simulink model "NumSim_standard_eVTOL"  (R2024b)
settings: Solver=ode14x  StartTime=0.0  StopTime=250  FixedStep=0.005  RelTol=1e-3
values from neighbouring files (symbols this model uses):
  aDl =     [initdata.mat]
  aDr =     [initdata.mat]
  aDyn =     [initdata.mat]
  Airport = init_airport('PHNL')    [initdata_HIL_eVTOL.m]
  aLat =     [initdata.mat]
  aLon =     [initdata.mat]
  D = Prop.D    [EOM_dt_MC.m]    (also in EOM_get_alf_dt_de_prop_evtol.m = CD * QS)
  dt0 = X(2)    [EOM_get_alf_dt_de_prop_evtol.m]    (also in initdata.mat = 0.258252593971; initdata_HIL_eVTOL.m = EOM_dt_MC)
  EAS0 = TAS0 / EAS2TAS    [initdata_HIL_eVTOL.m]
  FCS = init_FCS    [initdata_HIL_eVTOL.m]
  General = init_layoutdata    [EOM_dt_MC.m]    (also in build_optimized_CA.m; initdata.mat = ; initdata_HIL_eVTOL.m)
  h0 = Con(1)    [EOM_get_alf_dt_de_prop_evtol.m]    (also in initdata.mat = 450; initdata_HIL_eVTOL.m = 50)
  mass = Con(3)    [EOM_get_alf_dt_de_prop_evtol.m]    (also in initdata.mat = 2255.54; initdata_HIL_eVTOL.m = 7)
  Motor = init_motor_evtol    [EOM_dt_MC.m]    (also in initdata.mat = []; initdata_HIL_eVTOL.m)
  Prop = init_propeller_evtol_new    [EOM_dt_MC.m]    (also in initdata_HIL_eVTOL.m)
  R2D = 180/pi    (= 57.2957795131)    [EOM_get_alf_dt_de_prop_evtol.m]    (also in init_FCS.m; init_aerodata_evtol.m; init_airport.m; initdata.mat)
  theta0 = -0.0510981441662    [initdata.mat]
undefined symbols (not defined in the file or in its folder): A1, aDa, aDe, asbhl20env, B1, C1, de0, Earth, Environment, InitData, Kd, Kp, magnitude, Tc, WGS84
libraries: simulink_extras x26, simulink x18, slpidlib x14, vrlib x8, matrix_library x6, sharedutil x6, sharedtransform x5, aerolibwindfilters x4, aerolibatmos2 x3, aerolibobsolete x2, aerolibactuator x2, aerolibasang x2
(part 1 of 7)
settings Model: SimulationMode=accelerator  Creator=Administrator  LastModifiedBy=ZDB
settings SolverCC: EnableFixedStepZeroCrossing=on
settings OptimizationCC: ReuseModelBlockBuffer=off
settings DebuggingCC: UnconnectedInputMsg=warning  UnconnectedOutputMsg=warning  UnconnectedLineMsg=warning
settings ModelReferenceCC: EnableRefExpFcnMdlSchedulingChecks=on
settings RTWCC: GPUComputeCapability=3.5  DLArmComputeVersion=19.05

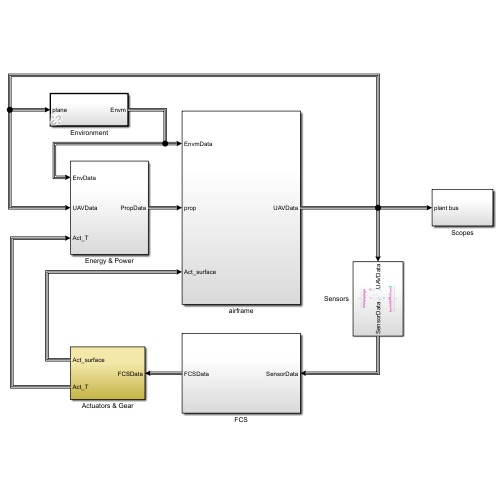
[thumbnail: Simulink's stored preview of the top-level diagram]
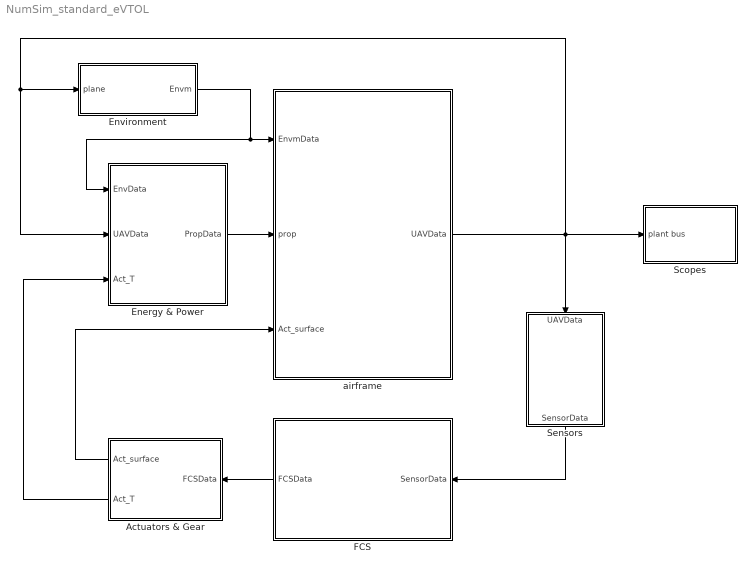
== system NumSim_standard_eVTOL ==
  Actuators & Gear : Subsystem
  Energy & Power : Subsystem
  Environment : Subsystem  AncestorBlock=asbhl20env/Environment  TreatAsAtomicUnit=on
      settings: LibrarySourceBlock=asbhl20env/Environment
  FCS : Subsystem
  Scopes : Subsystem
  Sensors : Subsystem
  airframe : Subsystem
  wires:
  Energy & Power/1(PropData) -> airframe/2(prop)
  Actuators & Gear/2(Act_T) -> Energy & Power/3(Act_T)
  airframe/1(UAVData) -> Energy & Power/2(UAVData), Environment/1(plane), Sensors/1(UAVData), Scopes/1(plant bus)
  Actuators & Gear/1(Act_surface) -> airframe/3(Act_surface)
  Environment/1(Envm) -> Energy & Power/1(EnvData), airframe/1(EnvmData)
  FCS/1(FCSData) -> Actuators & Gear/1(FCSData)
  Sensors/1(SensorData) -> FCS/1(SensorData)

== system NumSim_standard_eVTOL/Actuators & Gear ==
  FCSData : Inport
  Bus Creator : BusCreator  Inputs=3
  Bus Creator1 : BusCreator  Inputs=7
  Bus Selector : BusSelector  OutputSignals=ACTCMD.dl_cmd,ACTCMD.dt_final,ACTCMD.dr_cmd,ACTCMD.da_cmd,SensorData.Va,FCSCMD.icmd
  Demux : Demux  Outputs=6
  Gain{,1..11} (12 alike) : Gain
  Gain12 : Gain  Gain=57.3
  Max : MinMax  Function=max  Inputs=2
  Mux : Mux  Inputs=3
  Radians to Degrees1 : simulink_extras/Transformations/Radians to Degrees
  Radians to Degrees2 : simulink_extras/Transformations/Radians to Degrees
  Radians to Degrees3 : simulink_extras/Transformations/Radians to Degrees
  Rate Limiter : RateLimiter  RisingSlewLimit=0.12  FallingSlewLimit=-0.2  SampleTimeMode=inherited
  Saturation1 : Saturate  UpperLimit=25/57.3  LowerLimit=-25/57.3
  Saturation2 : Saturate  UpperLimit=25/57.3  LowerLimit=-25/57.3
  Saturation3 : Saturate  UpperLimit=25/57.3  LowerLimit=-25/57.3
  Scope : Scope
  Scope1 : Scope
  Scope3 : Scope
  Selector : Selector  InputPortWidth=3  IndexOptions=Index vector (dialog)  Indices=2  OutputSizes=1
  Selector1 : Selector  InputPortWidth=3  IndexOptions=Index vector (dialog)  Indices=3  OutputSizes=1
  Selector2 : Selector  InputPortWidth=3  IndexOptions=Index vector (dialog)  Indices=1  OutputSizes=1
  To Workspace : ToWorkspace  VariableName=i  SaveFormat=Timeseries  SampleTime=-1
  control output FW : Scope  NumInputPorts=3
  i : Constant  Commented=on  Value=0
  safe i_min : Lookup_n-D  NumberOfTableDimensions=1  BreakpointsForDimension1=[0,2,3.5,5,8,11,13,16,19,20,21, 22,30]  Table=[1.22,1.19,1.13,1.05,0.96,0.84,0.7,0.52,0.31,0.14,0.04,0,0]  InternalRulePriority=Speed  RndMeth=Simplest
  theta_b : Constant  Commented=on  Value=72.43773 * pi / 180
  Act_surface : Outport  VectorParamsAs1DForOutWhenUnconnected=off
  Act_T : Outport  Port=2  VectorParamsAs1DForOutWhenUnconnected=off
  tag scope: i=global
  wires:
  Mux/1 -> Selector2/1, Selector/1, Selector1/1
  Bus Creator/1 -> Act_surface/1
  Selector2/1 -> Gain6/1
  Saturation1/1 -> Gain3/1
  Saturation2/1 -> Radians to Degrees1/1, Bus Creator/2  "dr"
  Saturation3/1 -> Radians to Degrees2/1, Bus Creator/3  "da"
  Gain3/1 -> Radians to Degrees3/1, Bus Creator/1  "dl"
  Selector1/1 -> Gain1/1
  Selector/1 -> Gain/1
  Radians to Degrees3/1 -> control output FW/1  "da"
  Radians to Degrees1/1 -> control output FW/2  "de"
  Radians to Degrees2/1 -> control output FW/3  "dr"
  Gain/1 -> Gain4/1  "dr"
  Gain1/1 -> Gain5/1  "da"
  Gain4/1 -> Saturation2/1
  Gain5/1 -> Saturation3/1
  Bus Creator1/1 -> Act_T/1
  Gain6/1 -> Saturation1/1  "dl"
  FCSData/1 -> Bus Selector/1
  Bus Selector/1 -> Mux/1  "<dl_cmd>"
  Bus Selector/3 -> Mux/2  "<dr_cmd>"
  Bus Selector/4 -> Mux/3  "<da_cmd>"
  Gain2/1 -> Scope/1, Bus Creator1/1  "dt_1"
  Gain7/1 -> Scope3/1, Bus Creator1/2  "dt_2"
  Gain8/1 -> Bus Creator1/3  "dt_3"
  Gain9/1 -> Bus Creator1/4  "dt_4"
  Gain10/1 -> Bus Creator1/5  "dt_5"
  Gain11/1 -> Bus Creator1/6  "dt_6"
  Bus Selector/5 -> safe i_min/1  "<Va>"
  safe i_min/1 -> Max/2
  Max/1 -> Rate Limiter/1  "i"
  Bus Selector/6 -> Max/1  "<icmd>"
  Demux/1 -> Gain2/1
  Demux/2 -> Gain7/1
  Demux/3 -> Gain8/1
  Demux/4 -> Gain9/1
  Demux/5 -> Gain10/1
  Demux/6 -> Gain11/1
  Bus Selector/2 -> Demux/1  "<dt_final>"
  Rate Limiter/1 -> Gain12/1, Scope1/1, Bus Creator1/7, [i]  "i"
  Gain12/1 -> To Workspace/1

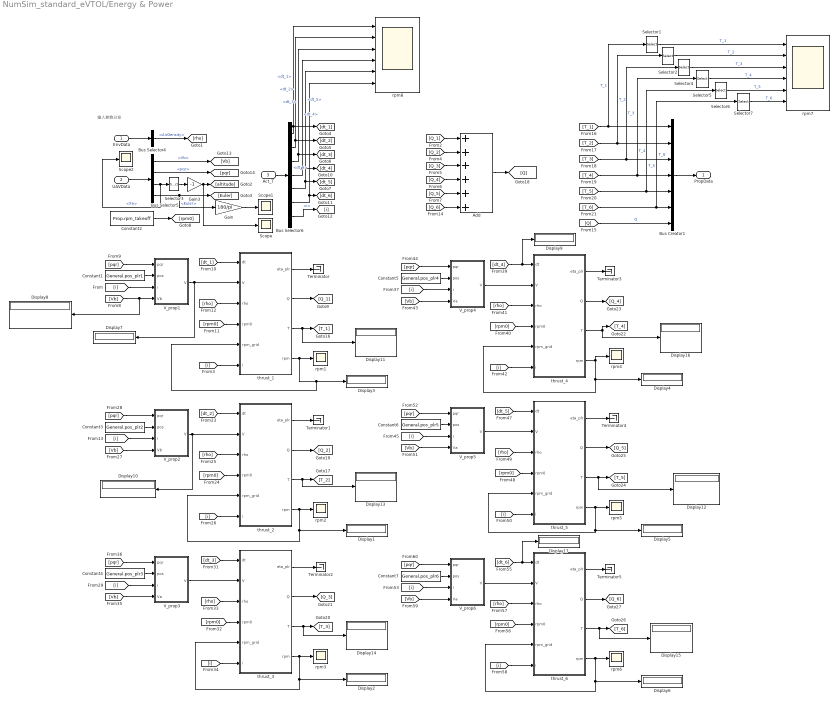
== system NumSim_standard_eVTOL/Energy & Power ==
  note: 输入参数分发
  EnvData : Inport
  UAVData : Inport  Port=2
  Act_T : Inport  Port=3
  Add : Sum  Inputs=++++++
  Bus Creator1 : BusCreator  Inputs=7
  Bus Selector4 : BusSelector  OutputSignals=AirDensity
  Bus Selector5 : BusSelector  OutputSignals=Vb,pqr,Xe,Euler
  Bus Selector6 : BusSelector  OutputSignals=dt_1,dt_2,dt_3,dt_4,dt_5,dt_6,i
  Constant1 : Constant  Value=General.pos_plr1
  Constant2 : Constant  Value=Prop.rpm_takeoff
  Constant3 : Constant  Value=General.pos_plr2
  Constant4 : Constant  Value=General.pos_plr3
  Constant5 : Constant  Value=General.pos_plr4
  Constant6 : Constant  Value=General.pos_plr5
  Constant7 : Constant  Value=General.pos_plr6
  Display{1..17} (17 alike) : Display
  Gain : Gain  Gain=180/pi
  Gain3 : Gain  Gain=-1
  Scope : Scope
  Scope1 : Scope
  Scope2 : Scope
  Selector{1..7} (7 alike) : Selector  InputPortWidth=3  IndexOptions=Index vector (dialog)  Indices=3  OutputSizes=1
  Terminator{,1..5} (6 alike) : Terminator
  V_prop1 : Subsystem
  V_prop2 : Subsystem
  V_prop3 : Subsystem
  V_prop4 : Subsystem
  V_prop5 : Subsystem
  V_prop6 : Subsystem
  rpm{1..6} (6 alike) : Scope
  rpm7 : Scope  NumInputPorts=6
  rpm8 : Scope  NumInputPorts=6
  thrust_1 : Subsystem
  thrust_2 : Subsystem
  thrust_3 : Subsystem
  thrust_4 : Subsystem
  thrust_5 : Subsystem
  thrust_6 : Subsystem
  PropData : Outport  VectorParamsAs1DForOutWhenUnconnected=off
  wires:
  Act_T/1 -> Bus Selector6/1
  [dt_1] -> thrust_1/1(dt)
  Constant1/1 -> V_prop1/2(pos)
  [rho] -> thrust_1/3(rho)
  [rpm0] -> thrust_1/4(rpm0)
  thrust_1/1(eta_plr) -> Terminator/1
  [pqr] -> V_prop1/1(pqr)
  [Vb] -> Display8/1, V_prop1/4(Vb)
  EnvData/1 -> Bus Selector4/1
  Bus Selector4/1 -> [rho]  "<AirDensity>"
  Bus Selector5/2 -> [pqr]  "<pqr>"
  Selector3/1 -> Gain3/1
  UAVData/1 -> Bus Selector5/1
  Bus Selector5/4 -> Gain/1, [Euler]  "<Euler>"
  Bus Selector5/1 -> [Vb]  "<Vb>"
  Bus Selector5/3 -> Scope2/1, Selector3/1  "<Xe>"
  Bus Selector6/1 -> rpm8/1, [dt_1]  "<dt_1>"
  Bus Selector6/5 -> [dt_5], rpm8/5  "<dt_5>"
  Bus Selector6/3 -> [dt_3], rpm8/3  "<dt_3>"
  Bus Selector6/2 -> [dt_2], rpm8/2  "<dt_2>"
  V_prop1/1(V) -> thrust_1/2(V), Display7/1
  [i] -> V_prop1/3(i)
  Constant2/1 -> [rpm0]
  thrust_1/4(rpm) -> thrust_1/5(rpm_grid), Display3/1, rpm1/1
  thrust_1/2(Q) -> [Q_1]
  Bus Selector6/4 -> [dt_4], rpm8/4  "<dt_4>"
  Bus Selector6/6 -> rpm8/6, [dt_6]  "<dt_6>"
  Bus Selector6/7 -> [i]  "<i>"
  [i] -> thrust_1/6(i)
  thrust_1/3(T) -> Display11/1, [T_1]
  [Q_1] -> Add/1
  [Q_6] -> Add/6
  [Q_5] -> Add/5
  [Q_4] -> Add/4
  [Q_3] -> Add/3
  [Q_2] -> Add/2
  Add/1 -> [Q]
  [Q] -> Bus Creator1/7  "Q"
  [T_1] -> Selector1/1, Bus Creator1/1  "T_1"
  [T_2] -> Selector2/1, Bus Creator1/2  "T_2"
  [T_3] -> Bus Creator1/3, Selector4/1  "T_3"
  [T_4] -> Bus Creator1/4, Selector5/1  "T_4"
  [T_5] -> Bus Creator1/5, Selector6/1  "T_5"
  [T_6] -> Bus Creator1/6, Selector7/1  "T_6"
  Bus Creator1/1 -> PropData/1
  thrust_2/4(rpm) -> rpm2/1, thrust_2/5(rpm_grid), Display1/1
  Constant3/1 -> V_prop2/2(pos)
  [dt_2] -> thrust_2/1(dt)
  V_prop2/1(V) -> Display10/1, thrust_2/2(V)
  thrust_2/2(Q) -> [Q_2]
  thrust_2/1(eta_plr) -> Terminator1/1
  [i] -> V_prop2/3(i)
  thrust_2/3(T) -> [T_2], Display13/1
  [rpm0] -> thrust_2/4(rpm0)
  [Vb] -> V_prop2/4(Vb)
  [pqr] -> V_prop2/1(pqr)
  [i] -> thrust_2/6(i)
  [rho] -> thrust_2/3(rho)
  [rho] -> thrust_3/3(rho)
  [pqr] -> V_prop3/1(pqr)
  [Vb] -> V_prop3/4(Va)
  [i] -> V_prop3/3(i)
  thrust_3/2(Q) -> [Q_3]
  V_prop3/1(V) -> thrust_3/2(V)
  [rpm0] -> thrust_3/4(rpm0)
  [dt_3] -> thrust_3/1(dt)
  thrust_3/4(rpm) -> thrust_3/5(rpm_grid), Display2/1, rpm3/1
  Constant4/1 -> V_prop3/2(pos)
  thrust_3/1(eta_plr) -> Terminator2/1
  [i] -> thrust_3/6(i)
  thrust_3/3(T) -> Display14/1, [T_3]
  [i] -> thrust_4/6(i)
  thrust_4/4(rpm) -> rpm4/1, thrust_4/5(rpm_grid), Display4/1
  Constant5/1 -> V_prop4/2(pos)
  thrust_4/1(eta_plr) -> Terminator3/1
  thrust_4/3(T) -> [T_4], Display16/1
  [dt_4] -> Display9/1, thrust_4/1(dt)
  V_prop4/1(V) -> thrust_4/2(V)
  [rpm0] -> thrust_4/4(rpm0)
  [i] -> V_prop4/3(i)
  [Vb] -> V_prop4/4(Va)
  [pqr] -> V_prop4/1(pqr)
  [rho] -> thrust_4/3(rho)
  thrust_4/2(Q) -> [Q_4]
  thrust_5/2(Q) -> [Q_5]
  thrust_5/3(T) -> Display12/1, [T_5]
  [rho] -> thrust_5/3(rho)
  [pqr] -> V_prop5/1(pqr)
  [rpm0] -> thrust_5/4(rpm0)
  Constant6/1 -> V_prop5/2(pos)
  thrust_5/1(eta_plr) -> Terminator4/1
  [dt_5] -> thrust_5/1(dt)
  [i] -> V_prop5/3(i)
  V_prop5/1(V) -> thrust_5/2(V)
  [i] -> thrust_5/6(i)
  thrust_5/4(rpm) -> thrust_5/5(rpm_grid), Display5/1, rpm5/1
  [Vb] -> V_prop5/4(Va)
  [i] -> V_prop6/3(i)
  [Vb] -> V_prop6/4(Va)
  thrust_6/1(eta_plr) -> Terminator5/1
  V_prop6/1(V) -> thrust_6/2(V)
  [dt_6] -> Display17/1, thrust_6/1(dt)
  thrust_6/4(rpm) -> thrust_6/5(rpm_grid), Display6/1, rpm6/1
  thrust_6/2(Q) -> [Q_6]
  thrust_6/3(T) -> Display15/1, [T_6]
  Constant7/1 -> V_prop6/2(pos)
  [rho] -> thrust_6/3(rho)
  [pqr] -> V_prop6/1(pqr)
  [rpm0] -> thrust_6/4(rpm0)
  [i] -> thrust_6/6(i)
  Selector1/1 -> rpm7/1  "T_1"
  Selector2/1 -> rpm7/2  "T_2"
  Selector4/1 -> rpm7/3  "T_3"
  Selector5/1 -> rpm7/4  "T_4"
  Selector6/1 -> rpm7/5  "T_5"
  Selector7/1 -> rpm7/6  "T_6"
  Gain3/1 -> Scope/1, [altitude]
  Gain/1 -> Scope1/1

== system NumSim_standard_eVTOL/Environment ==
  plane : Inport
  Bus Creator : BusCreator  Inputs=8
  Bus Selector : BusSelector  OutputSignals=Xe,Ve,DCM_be
  COESA Atmosphere Model : aerolibatmos2/COESA Atmosphere Model  units=Metric (MKS)  spec=1976 COESA-extended U.S. Standard Atmosphere  model=Profile  profile_var=High temperature  profile_percent=1%  profile_alt=5 km (16404 ft)  envelope_var=High temperature  envelope_percent=1%  action=Warning
  Height : Selector  InputPortWidth=3  IndexOptions=Index vector (dialog)  Indices=[3]  OutputSizes=1
  Latitude : Constant  Value=40
  Terrain : Subsystem
  WGS84 Gravity Model : aerolibobsolete/WGS84 Gravity Model  model=WGS84 Taylor Series  units=Metric (MKS)  no_atmos=on  precessing=on  month=February  day=1  year=2000  no_centrifugal=on  action=None
  Wind Models : Subsystem
  x : Selector  InputPortWidth=3  IndexOptions=Index vector (dialog)  Indices=1  OutputSizes=1
  z-->h : Abs
  Envm : Outport  InitialOutput=0  VectorParamsAs1DForOutWhenUnconnected=off
  wires:
  COESA Atmosphere Model/4 -> Bus Creator/7  "AirDensity"
  COESA Atmosphere Model/2 -> Bus Creator/5  "a"
  COESA Atmosphere Model/3 -> Bus Creator/6  "Po"
  COESA Atmosphere Model/1 -> Bus Creator/4  "To"
  Height/1 -> z-->h/1
  Bus Creator/1 -> Envm/1  "EnvmData"
  plane/1 -> Bus Selector/1
  z-->h/1 -> COESA Atmosphere Model/1, WGS84 Gravity Model/1, Wind Models/3(Altitude)
  Bus Selector/1 -> x/1, Terrain/1(Xe), Height/1  "<Xe>"
  Bus Selector/2 -> Wind Models/2(Ve)  "<Ve>"
  Bus Selector/3 -> Wind Models/4(DCM)  "<DCM_be>"
  Latitude/1 -> WGS84 Gravity Model/2
  WGS84 Gravity Model/1 -> Bus Creator/8  "g"
  Terrain/1(hground) -> Bus Creator/1  "hground"
  Wind Models/1(ug,vg,wg1) -> Bus Creator/2
  Wind Models/2(pg,qg,rg1) -> Bus Creator/3
  x/1 -> Wind Models/1(Xe_x)

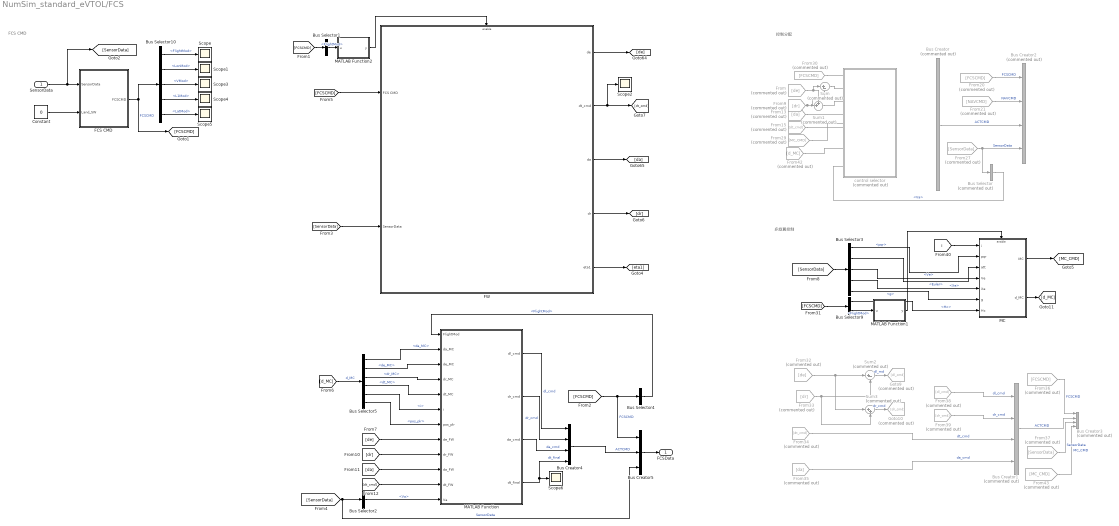
== system NumSim_standard_eVTOL/FCS ==
  note: 控制分配
  note: 多旋翼控制
  note: FCS CMD
  SensorData : Inport
  Bus Creator{,1..3} (4 alike) : BusCreator  Commented=on  Inputs=4
  Bus Creator4 : BusCreator  Inputs=4
  Bus Creator5 : BusCreator  Inputs=3
  Bus Selector : BusSelector  Commented=on  OutputSignals=Va
  Bus Selector1 : BusSelector  OutputSignals=FlightMod
  Bus Selector10 : BusSelector  OutputSignals=FlightMod,LonMod,VMod,L1Mod,LatMod
  Bus Selector2 : BusSelector  OutputSignals=Va
  Bus Selector3 : BusSelector  OutputSignals=pqr,Euler,Ve,Xe,g
  Bus Selector4 : BusSelector  OutputSignals=FlightMod
  Bus Selector5 : BusSelector  OutputSignals=da_MC,de_MC,dr_MC,dt_MC,i,pos_plr
  Bus Selector9 : BusSelector  OutputSignals=Hc,FlightMod
  Constant : Constant  Value=0
  FCS CMD : Subsystem
  FW : Subsystem
  From : From  Commented=on  GotoTag=de
  From13 : From  Commented=on  GotoTag=da
  From15 : From  Commented=on  GotoTag=dt_cmd
  From20 : From  Commented=on  GotoTag=FCSCMD
      settings: CloseFcn=tagdialog Close
  From21 : From  Commented=on  GotoTag=NAVCMD
      settings: CloseFcn=tagdialog Close
  From27 : From  Commented=on  GotoTag=SensorData
  From29 : From  Commented=on  GotoTag=MC_CMD
  From30 : From  Commented=on  GotoTag=FCSCMD
      settings: CloseFcn=tagdialog Close
  From32 : From  Commented=on  GotoTag=de
  From33 : From  Commented=on  GotoTag=dr
  From34 : From  Commented=on  GotoTag=dt_cmd
  From35 : From  Commented=on  GotoTag=da
  From36 : From  Commented=on  GotoTag=FCSCMD
  From37 : From  Commented=on  GotoTag=SensorData
  From38 : From  Commented=on  GotoTag=dl_cmd
  From39 : From  Commented=on  GotoTag=dr_cmd
  From42 : From  Commented=on  GotoTag=d_MC
  From43 : From  Commented=on  GotoTag=MC_CMD
  From9 : From  Commented=on  GotoTag=dr
  Goto10 : Goto  Commented=on  GotoTag=dr_cmd
  Goto9 : Goto  Commented=on  GotoTag=dl_cmd
  MATLAB Function : MATLAB Function  TreatAsAtomicUnit=on
  MATLAB Function1 : MATLAB Function  TreatAsAtomicUnit=on
  MATLAB Function2 : MATLAB Function  TreatAsAtomicUnit=on
  MC : Subsystem
  Scope{,1..6} (7 alike) : Scope
  Sum : Sum  Commented=on  Inputs=|+-
  Sum1 : Sum  Commented=on  Inputs=++|
  Sum2 : Sum  Commented=on  Inputs=|+-
  Sum3 : Sum  Commented=on  Inputs=|++
  control selector : Subsystem  Commented=on
  FCSData : Outport  VectorParamsAs1DForOutWhenUnconnected=off
  wires:
  Bus Creator/1 -> Bus Creator2/3  "ACTCMD"
  SensorData/1 -> FCS CMD/1(SensorData), [SensorData]
  FCS CMD/1(FCSCMD) -> Bus Selector10/1, [FCSCMD]  "FCSCMD"
  From20/1 -> Bus Creator2/1  "FCSCMD"
  From21/1 -> Bus Creator2/2  "NAVCMD"
  From30/1 -> ?
  [SensorData] -> Bus Selector3/1
  Bus Selector3/1 -> MC/2(pqr)  "<pqr>"
  Bus Selector3/2 -> MC/3(att)  "<Euler>"
  Bus Selector3/3 -> MC/4(Ve)  "<Ve>"
  Bus Selector3/4 -> MC/5(Xe)  "<Xe>"
  Constant/1 -> FCS CMD/2(Land_SW)
  MC/1(MC) -> [MC_CMD]
  Bus Selector3/5 -> MC/6(g)  "<g>"
  From/1 -> Sum1/1, Sum/1
  From9/1 -> Sum/2, Sum1/2
  Sum/1 -> ?
  Sum1/1 -> ?
  From13/1 -> ?
  From15/1 -> ?
  From27/1 -> Bus Selector/1, Bus Creator2/4  "SensorData"
  From29/1 -> ?
  Bus Selector/1 -> ?  "<Va>"
  [FCSCMD] -> Bus Selector9/1
  Bus Selector9/1 -> MC/7(Hc)  "<Hc>"
  Bus Selector10/1 -> Scope/1  "<FlightMod>"
  Bus Selector10/2 -> Scope1/1  "<LonMod>"
  Bus Selector10/3 -> Scope3/1  "<VMod>"
  Bus Selector10/4 -> Scope4/1  "<L1Mod>"
  Bus Selector10/5 -> Scope5/1  "<LatMod>"
  From33/1 -> Sum3/2, Sum2/2
  From32/1 -> Sum3/1, Sum2/1
  From34/1 -> Bus Creator1/3  "dt_cmd"
  From35/1 -> Bus Creator1/4  "da_cmd"
  Bus Creator1/1 -> Bus Creator3/2  "ACTCMD"
  From36/1 -> Bus Creator3/1  "FCSCMD"
  From37/1 -> Bus Creator3/3  "SensorData"
  Sum2/1 -> Goto9/1  "dl_md"
  Sum3/1 -> Goto10/1  "dr_cmd"
  From39/1 -> Bus Creator1/2  "dr_cmd"
  From38/1 -> Bus Creator1/1  "dl_cmd"
  Bus Selector9/2 -> MATLAB Function1/1(u)  "<FlightMod>"
  [i] -> MC/1(i)
  MC/2(d_MC) -> [d_MC]
  From42/1 -> ?
  ? -> Bus Creator/1  "dl_cmd"
  ? -> Bus Creator/2  "dr_cmd"
  ? -> Bus Creator/3  "da_cmd"
  ? -> Bus Creator/4  "dt_cmd"
  From43/1 -> Bus Creator3/4  "MC_CMD"
  FW/1(de) -> [de]
  [FCSCMD] -> FW/1(FCS CMD)
  [SensorData] -> FW/2(SensorData)
  FW/5(eta1) -> [eta1]
  FW/4(dr) -> [dr]
  FW/3(da) -> [da]
  FW/2(dt_cmd) -> Scope2/1, [dt_cmd]
  [FCSCMD] -> Bus Selector1/1
  Bus Selector1/1 -> MATLAB Function2/1(u)  "<FlightMod>"
  MATLAB Function2/1(y) -> FW/Enable
  MATLAB Function/1(dl_cmd) -> Bus Creator4/1  "dl_cmd"
  MATLAB Function/2(dr_cmd) -> Bus Creator4/2  "dr_cmd"
  MATLAB Function/3(da_cmd) -> Bus Creator4/3  "da_cmd"
  MATLAB Function/4(dt_final) -> Scope6/1, Bus Creator4/4  "dt_final"
  Bus Creator4/1 -> Bus Creator5/2  "ACTCMD"
  [SensorData] -> Bus Creator5/3, Bus Selector2/1  "SensorData"
  Bus Selector2/1 -> MATLAB Function/12(Va)  "<Va>"
  [FCSCMD] -> Bus Selector4/1, Bus Creator5/1  "FCSCMD"
  Bus Creator5/1 -> FCSData/1
  Bus Selector4/1 -> MATLAB Function/1(FlightMod)  "<FlightMod>"
  [d_MC] -> Bus Selector5/1  "d_MC"
  Bus Selector5/6 -> MATLAB Function/7(pos_plr)  "<pos_plr>"
  Bus Selector5/1 -> MATLAB Function/2(da_MC)  "<da_MC>"
  Bus Selector5/2 -> MATLAB Function/3(de_MC)  "<de_MC>"
  Bus Selector5/3 -> MATLAB Function/4(dr_MC)  "<dr_MC>"
  Bus Selector5/4 -> MATLAB Function/5(dt_MC)  "<dt_MC>"
  Bus Selector5/5 -> MATLAB Function/6(i)  "<i>"
  [de] -> MATLAB Function/8(de_FW)
  [dr] -> MATLAB Function/9(dr_FW)
  [da] -> MATLAB Function/10(da_FW)
  [dt_cmd] -> MATLAB Function/11(dt_FW)
  MATLAB Function1/1(y) -> MC/Enable

== system NumSim_standard_eVTOL/Scopes ==
  plant bus : Inport
  {1,6..7,14} (4 alike) : Selector  InputPortWidth=3  IndexOptions=Index vector (dialog)  Indices=2  OutputSizes=1
  {3..4,10..11} (4 alike) : Selector  InputPortWidth=3  IndexOptions=Index vector (dialog)  Indices=3  OutputSizes=1
  {2,5,8..9} (4 alike) : Selector  InputPortWidth=3  IndexOptions=Index vector (dialog)  Indices=1  OutputSizes=1
  Bus Selector : BusSelector  OutputSignals=Euler,Ve,Xe,Va,alpha,beta,pqr,gamma,Ab
  Gain : Gain  Gain=-1
  Radians to Degrees{,1,3..5} (5 alike) : simulink_extras/Transformations/Radians to Degrees
  To Workspace : ToWorkspace  VariableName=x  SaveFormat=Timeseries  SampleTime=-1
  To Workspace1 : ToWorkspace  VariableName=Va  SaveFormat=Timeseries  SampleTime=-1
  To Workspace2 : ToWorkspace  VariableName=height  SaveFormat=Timeseries  SampleTime=-1
  Va : Scope
  Ve : Scope
  alpha : Scope
  ax : Scope
  ay : Scope
  az : Scope
  beta : Scope
  gamma : Scope
  height : Scope
  p : Scope
  phi : Scope
  psi : Scope
  q : Scope
  r : Scope
  theta : Scope
  x : Scope
  y : Scope
  wires:
  Radians to Degrees5/1 -> [Euler]
  plant bus/1 -> Bus Selector/1
  1/1 -> theta/1  "theta(deg)"
  Bus Selector/3 -> [Xe]  "<Xe>"
  2/1 -> phi/1  "phi(deg)"
  4/1 -> psi/1  "psi(deg)"
  Bus Selector/5 -> Radians to Degrees/1  "<alpha>"
  [Euler] -> 1/1, 2/1, 4/1
  Bus Selector/1 -> Radians to Degrees5/1  "<Euler>"
  [Xe] -> 5/1, 14/1, 11/1
  Bus Selector/2 -> [Ve]  "<Ve>"
  Bus Selector/4 -> [V]  "<Va>"
  Radians to Degrees/1 -> [alpha]
  Bus Selector/6 -> Radians to Degrees3/1  "<beta>"
  Radians to Degrees3/1 -> [beta]
  [beta] -> beta/1  "beta(deg)"
  [alpha] -> alpha/1  "alpha(deg)"
  [Ve] -> Ve/1  "Ve(m/s)"
  Bus Selector/7 -> Radians to Degrees1/1  "<pqr>"
  6/1 -> q/1  "q(deg/s)"
  9/1 -> p/1  "p(deg/s)"
  10/1 -> r/1  "r(deg/s)"
  [pqr] -> 10/1, 9/1, 6/1
  Radians to Degrees1/1 -> [pqr]
  11/1 -> Gain/1
  Gain/1 -> To Workspace2/1, height/1  "h(m)"
  5/1 -> To Workspace/1, x/1  "x(m)"
  Bus Selector/8 -> Radians to Degrees4/1  "<gamma>"
  Radians to Degrees4/1 -> [gamma]
  [gamma] -> gamma/1  "\\gamma (deg)"
  14/1 -> y/1  "y(m)"
  [V] -> To Workspace1/1, Va/1  "Va(m/s)"
  Bus Selector/9 -> [Ab]  "<Ab>"
  [Ab] -> 8/1, 7/1, 3/1
  3/1 -> az/1  "az"
  8/1 -> ax/1  "ax"
  7/1 -> ay/1  "ay"

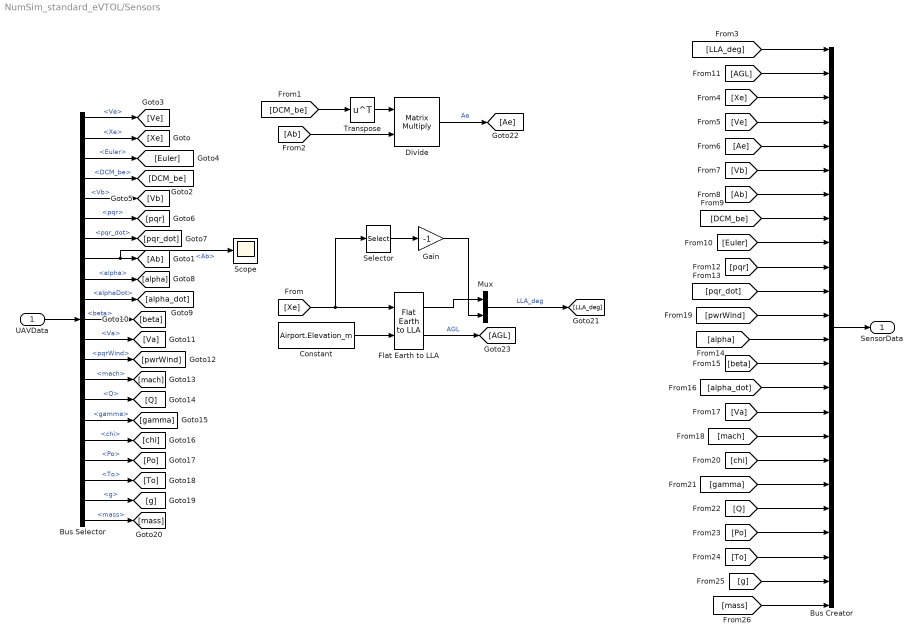
== system NumSim_standard_eVTOL/Sensors ==
  UAVData : Inport
  Bus Creator : BusCreator  Inputs=24
  Bus Selector : BusSelector  OutputSignals=Ve,Xe,Euler,DCM_be,Vb,pqr,pqr_dot,Ab,alpha,alphaDot,beta,Va,pqrWind,mach,Q,gamma,chi,Po,To,g,mass
  Constant : Constant  Value=Airport.Elevation_m
  Divide : Product  Inputs=**  Multiplication=Matrix(*)
  Flat Earth to LLA : aerolibtransform2/Flat Earth to LLA  units=Metric (MKS)  ptype=Earth (WGS84)  F=1/298.257223563  R=6378137  refPosPort=off  LL0=InitData.LLA(1:2)*R2D  psi=0
  Gain : Gain  Gain=-1
  Mux : Mux  Inputs=2
  Scope : Scope
  Selector : Selector  InputPortWidth=3  IndexOptions=Index vector (dialog)  Indices=3  OutputSizes=1
  Transpose : Math  Operator=transpose
  SensorData : Outport
  wires:
  Constant/1 -> Flat Earth to LLA/2
  Flat Earth to LLA/1 -> Mux/1
  Flat Earth to LLA/2 -> [AGL]  "AGL"
  UAVData/1 -> Bus Selector/1
  Bus Selector/2 -> [Xe]  "<Xe>"
  [Xe] -> Selector/1, Flat Earth to LLA/1
  Bus Selector/8 -> Scope/1, [Ab]  "<Ab>"
  Bus Selector/4 -> [DCM_be]  "<DCM_be>"
  [DCM_be] -> Transpose/1
  [Ab] -> Divide/2
  Selector/1 -> Gain/1
  Gain/1 -> Mux/2
  Mux/1 -> [LLA_deg]  "LLA_deg"
  Bus Selector/1 -> [Ve]  "<Ve>"
  Bus Selector/3 -> [Euler]  "<Euler>"
  Bus Selector/5 -> [Vb]  "<Vb>"
  Bus Selector/6 -> [pqr]  "<pqr>"
  Bus Selector/7 -> [pqr_dot]  "<pqr_dot>"
  Bus Selector/9 -> [alpha]  "<alpha>"
  Bus Selector/10 -> [alpha_dot]  "<alphaDot>"
  Bus Selector/11 -> [beta]  "<beta>"
  Bus Selector/12 -> [Va]  "<Va>"
  Bus Selector/13 -> [pwrWind]  "<pqrWind>"
  Bus Selector/14 -> [mach]  "<mach>"
  Bus Selector/15 -> [Q]  "<Q>"
  Bus Selector/16 -> [gamma]  "<gamma>"
  Bus Selector/17 -> [chi]  "<chi>"
  Bus Selector/18 -> [Po]  "<Po>"
  Bus Selector/19 -> [To]  "<To>"
  Bus Selector/20 -> [g]  "<g>"
  Bus Selector/21 -> [mass]  "<mass>"
  Transpose/1 -> Divide/1
  Divide/1 -> [Ae]  "Ae"
  [LLA_deg] -> Bus Creator/1
  [Xe] -> Bus Creator/3
  [Ve] -> Bus Creator/4
  [Ae] -> Bus Creator/5
  [Vb] -> Bus Creator/6
  [Ab] -> Bus Creator/7
  [DCM_be] -> Bus Creator/8
  [Euler] -> Bus Creator/9
  [AGL] -> Bus Creator/2
  [pqr] -> Bus Creator/10
  [pqr_dot] -> Bus Creator/11
  [alpha] -> Bus Creator/13
  [beta] -> Bus Creator/14
  [alpha_dot] -> Bus Creator/15
  [Va] -> Bus Creator/16
  [mach] -> Bus Creator/17
  [pwrWind] -> Bus Creator/12
  [chi] -> Bus Creator/18
  [gamma] -> Bus Creator/19
  [Q] -> Bus Creator/20
  [Po] -> Bus Creator/21
  [To] -> Bus Creator/22
  [g] -> Bus Creator/23
  [mass] -> Bus Creator/24
  Bus Creator/1 -> SensorData/1

== system NumSim_standard_eVTOL/airframe ==
  EnvmData : Inport
  prop : Inport  Port=2
  Act_surface : Inport  Port=3
  6DoF (Euler Angles)1 : aerolibobsolete/6DoF (Euler Angles)  units=Metric (MKS)  mtype=Fixed  rep=Euler Angles  xme_0=InitData.Xe  Vm_0=InitData.Vb  eul_0=InitData.Euler+[0,0,0]/57.3  pm_0=InitData.pqr  mass_0=InitData.mass0  mass_e=0.5  mass_f=2.0  inertia=Mass.Inertial  inertia_e=eye(3)  inertia_f=2*eye(3)  k_quat=1.0
  Bus Creator : BusCreator  Inputs=21
  Constant3 : Constant  Value=mass
  Flight Conditions : Subsystem  AncestorBlock=asbhl20vehicle/Vehicle/Aerodynamic/DerivedConditions
      settings: LibrarySourceBlock=asbhl20vehicle/Vehicle/Aerodynamic/DerivedConditions
  Fly : Constant
  Gain : Gain  Gain=[1,1,1]
  Gain1 : Gain  Gain=[1,1,1]
  Manual Switch : ManualSwitch
  Product : Product
  Product1 : Product
  force moment : Subsystem
  init : Constant  Value=0
  UAVData : Outport  VectorParamsAs1DForOutWhenUnconnected=off
  wires:
  prop/1 -> force moment/3(prop)
  6DoF (Euler Angles)1/1 -> Bus Creator/1  "Ve"
  6DoF (Euler Angles)1/2 -> Bus Creator/2  "Xe"
  6DoF (Euler Angles)1/8 -> Bus Creator/8  "Ab"
  6DoF (Euler Angles)1/7 -> Bus Creator/7  "pqr_dot"
  6DoF (Euler Angles)1/6 -> Bus Creator/6  "pqr"
  6DoF (Euler Angles)1/5 -> Bus Creator/5  "Vb"
  Act_surface/1 -> force moment/2(Act_surface)
  Bus Creator/1 -> Flight Conditions/2(PlantData), force moment/1(PlantData), UAVData/1  "UAVData"
  EnvmData/1 -> Flight Conditions/1(EnvmData), force moment/4(EnvmData)
  Flight Conditions/1(Alpha) -> Bus Creator/9  "alpha"
  Flight Conditions/3(Beta) -> Bus Creator/11  "beta"
  Flight Conditions/4(V) -> Bus Creator/12  "Va"
  Flight Conditions/5(pqrWind) -> Bus Creator/13  "pqrWind"
  Flight Conditions/6(Mach) -> Bus Creator/14  "mach"
  Flight Conditions/7(Qbar) -> Bus Creator/15  "Q"
  Flight Conditions/8(gamma) -> Bus Creator/16  "gamma"
  Flight Conditions/2(AlphaDot) -> Bus Creator/10  "alphaDot"
  6DoF (Euler Angles)1/4 -> Bus Creator/4  "DCM_be"
  Constant3/1 -> Bus Creator/21  "mass"
  Flight Conditions/9(chi) -> Bus Creator/17  "chi"
  Flight Conditions/10(Po) -> Bus Creator/18  "Po"
  Flight Conditions/11(To) -> Bus Creator/19  "To"
  Flight Conditions/12(g) -> Bus Creator/20  "g"
  force moment/1(Fb (X Y Z)) -> Gain/1
  force moment/2(M (L M N)) -> Gain1/1
  6DoF (Euler Angles)1/3 -> Bus Creator/3  "Euler"
  Product/1 -> 6DoF (Euler Angles)1/1
  Gain1/1 -> Product1/2
  Product1/1 -> 6DoF (Euler Angles)1/2
  Gain/1 -> Product/2
  Fly/1 -> Manual Switch/1
  init/1 -> Manual Switch/2
  Manual Switch/1 -> Product1/1, Product/1  "是否关闭力输出"

== system NumSim_standard_eVTOL/Energy & Power/V_prop1 ==
  note: 将速度矢量投影到桨轴
  pqr : Inport
  pos : Inport  Port=2
  i : Inport  Port=3
  Vb : Inport  Port=4
  Cross Product4 : matrix_library/Cross Product
  Display1 : Display
  Display2 : Display
  Display8 : Display
  Sum2 : Sum  Inputs=|++
  v_b to v_prop : Subsystem
  V : Outport
  wires:
  pos/1 -> Cross Product4/2
  pqr/1 -> Cross Product4/1
  Vb/1 -> Display2/1, Sum2/2
  i/1 -> v_b to v_prop/2(i)
  Cross Product4/1 -> Display8/1, Sum2/1
  Sum2/1 -> Display1/1, v_b to v_prop/1(V_body)
  v_b to v_prop/1(V) -> V/1

== system NumSim_standard_eVTOL/Energy & Power/V_prop2 ==
  note: 将速度矢量投影到桨轴
  pqr : Inport
  pos : Inport  Port=2
  i : Inport  Port=3
  Vb : Inport  Port=4
  Cross Product4 : matrix_library/Cross Product
  Sum2 : Sum  Inputs=|++
  v_b to v_prop : Subsystem
  V : Outport
  wires:
  pos/1 -> Cross Product4/2
  pqr/1 -> Cross Product4/1
  Vb/1 -> Sum2/2
  i/1 -> v_b to v_prop/2(i)
  Cross Product4/1 -> Sum2/1
  Sum2/1 -> v_b to v_prop/1(V_body)
  v_b to v_prop/1(V) -> V/1

== system NumSim_standard_eVTOL/Energy & Power/V_prop3 ==
  note: 将速度矢量投影到桨轴
  pqr : Inport
  pos : Inport  Port=2
  i : Inport  Port=3
  Va : Inport  Port=4
  Cross Product4 : matrix_library/Cross Product
  Sum2 : Sum  Inputs=|++
  v_b to v_prop : Subsystem
  V : Outport
  wires:
  pos/1 -> Cross Product4/2
  pqr/1 -> Cross Product4/1
  Va/1 -> Sum2/2
  i/1 -> v_b to v_prop/2(i)
  Cross Product4/1 -> Sum2/1
  Sum2/1 -> v_b to v_prop/1(V_body)
  v_b to v_prop/1(V) -> V/1

== system NumSim_standard_eVTOL/Energy & Power/V_prop4 ==
  note: 将速度矢量投影到桨轴
  pqr : Inport
  pos : Inport  Port=2
  i : Inport  Port=3
  Va : Inport  Port=4
  Cross Product4 : matrix_library/Cross Product
  Sum2 : Sum  Inputs=|++
  v_b to v_prop : Subsystem
  V : Outport
  wires:
  pos/1 -> Cross Product4/2
  pqr/1 -> Cross Product4/1
  Va/1 -> Sum2/2
  i/1 -> v_b to v_prop/2(i)
  Cross Product4/1 -> Sum2/1
  Sum2/1 -> v_b to v_prop/1(V_body)
  v_b to v_prop/1(V) -> V/1

== system NumSim_standard_eVTOL/Energy & Power/V_prop5 ==
  note: 将速度矢量投影到桨轴
  pqr : Inport
  pos : Inport  Port=2
  i : Inport  Port=3
  Va : Inport  Port=4
  Cross Product4 : matrix_library/Cross Product
  Sum2 : Sum  Inputs=|++
  v_b to v_prop : Subsystem
  V : Outport
  wires:
  pos/1 -> Cross Product4/2
  pqr/1 -> Cross Product4/1
  Va/1 -> Sum2/2
  i/1 -> v_b to v_prop/2(i)
  Cross Product4/1 -> Sum2/1
  Sum2/1 -> v_b to v_prop/1(V_body)
  v_b to v_prop/1(V) -> V/1

== system NumSim_standard_eVTOL/Energy & Power/V_prop6 ==
  note: 将速度矢量投影到桨轴
  pqr : Inport
  pos : Inport  Port=2
  i : Inport  Port=3
  Va : Inport  Port=4
  Cross Product4 : matrix_library/Cross Product
  Sum2 : Sum  Inputs=|++
  v_b to v_prop : Subsystem
  V : Outport
  wires:
  pos/1 -> Cross Product4/2
  pqr/1 -> Cross Product4/1
  Va/1 -> Sum2/2
  i/1 -> v_b to v_prop/2(i)
  Cross Product4/1 -> Sum2/1
  Sum2/1 -> v_b to v_prop/1(V_body)
  v_b to v_prop/1(V) -> V/1

== system NumSim_standard_eVTOL/Energy & Power/thrust_1 ==
  note: 将推力、扭矩按电机倾转角转化为向量
  note: 求桨的推力、扭矩、功率、效率
  dt : Inport
  V : Inport  Port=2
  rho : Inport  Port=3
  rpm0 : Inport  Port=4
  rpm_grid : Inport  Port=5
  i : Inport  Port=6
  Constant : Constant  Commented=on  Value=2.5
  Gain2 : Gain  Gain=-1
  Gain4 : Gain  Gain=pi/30
  Manual Switch : ManualSwitch  Commented=on  CurrentSetting=0
  Motor : Subsystem
  Mux1 : Mux  Inputs=2
  Mux2 : Mux  Inputs=3
  Mux3 : Mux  Inputs=2
  Mux4 : Mux  Inputs=3
  Product : Product  Inputs=*/
  "Propeller " : Subsystem
  Q_x : Fcn  Expr=-u[1]*cos(u[2])
  Q_y : Fcn  Expr=0
  Q_z : Fcn  Expr=u[1]*sin(u[2])
  Saturation : Saturate  UpperLimit=inf  LowerLimit=1
  T_x : Fcn  Expr=u[1]*cos(u[2])
  T_y : Fcn  Expr=0
  T_z : Fcn  Expr=-u[1]*sin(u[2])
  eta_plr : Outport  VectorParamsAs1DForOutWhenUnconnected=off
  Q : Outport  Port=2
  T : Outport  Port=3  VectorParamsAs1DForOutWhenUnconnected=off
  rpm : Outport  Port=4  VectorParamsAs1DForOutWhenUnconnected=off
  wires:
  Saturation/1 -> Motor/4(rpm0)
  rpm0/1 -> Saturation/1
  "Propeller "/2(T (N)) -> [T]
  dt/1 -> Motor/2(dt)
  Motor/1(rpm) -> rpm/1, Gain4/1, "Propeller "/1(rpm)
  "Propeller "/3(eta_p) -> eta_plr/1
  rho/1 -> [rho]
  "Propeller "/1(P_plr (w)) -> Motor/1(P_shaft), Product/1
  Gain4/1 -> Product/2  "omega"
  Product/1 -> Gain2/1
  T_y/1 -> Mux2/2
  Mux1/1 -> T_z/1, T_x/1, T_y/1
  T_x/1 -> Mux2/1
  i/1 -> [i]
  T_z/1 -> Mux2/3
  Mux2/1 -> T/1
  [T] -> Mux1/1
  Mux4/1 -> Q/1
  [i] -> Mux3/2
  Q_z/1 -> Mux4/3
  Q_x/1 -> Mux4/1
  Mux3/1 -> Q_z/1, Q_x/1, Q_y/1
  Q_y/1 -> Mux4/2
  [Q] -> Mux3/1
  [i] -> Mux1/2
  Gain2/1 -> [Q]
  [V] -> Motor/3(V)
  [V] -> "Propeller "/2(V)
  [rho] -> Motor/5(rho)
  [rho] -> "Propeller "/3(rho)
  Constant/1 -> Manual Switch/1
  V/1 -> [V]
  rpm_grid/1 -> Motor/6(rpm_grid)

== system NumSim_standard_eVTOL/Energy & Power/thrust_2 ==
  note: 将推力、扭矩按电机倾转角转化为向量
  note: 求桨的推力、扭矩、功率、效率
  dt : Inport
  V : Inport  Port=2
  rho : Inport  Port=3
  rpm0 : Inport  Port=4
  rpm_grid : Inport  Port=5
  i : Inport  Port=6
  Constant : Constant  Commented=on  Value=2.5
  Gain4 : Gain  Gain=pi/30
  Manual Switch : ManualSwitch  Commented=on  CurrentSetting=0
  Motor : Subsystem
  Mux1 : Mux  Inputs=2
  Mux2 : Mux  Inputs=3
  Mux3 : Mux  Inputs=2
  Mux4 : Mux  Inputs=3
  Product : Product  Inputs=*/
  "Propeller " : Subsystem
  Q_x : Fcn  Expr=-u[1]*cos(u[2])
  Q_y : Fcn  Expr=0
  Q_z : Fcn  Expr=u[1]*sin(u[2])
  Saturation : Saturate  UpperLimit=inf  LowerLimit=1
  T_x : Fcn  Expr=u[1]*cos(u[2])
  T_y : Fcn  Expr=0
  T_z : Fcn  Expr=-u[1]*sin(u[2])
  eta_plr : Outport  VectorParamsAs1DForOutWhenUnconnected=off
  Q : Outport  Port=2
  T : Outport  Port=3  VectorParamsAs1DForOutWhenUnconnected=off
  rpm : Outport  Port=4  VectorParamsAs1DForOutWhenUnconnected=off
  wires:
  Saturation/1 -> Motor/4(rpm0)
  rpm0/1 -> Saturation/1
  "Propeller "/2(T (N)) -> [T]
  dt/1 -> Motor/2(dt)
  Motor/1(rpm) -> rpm/1, Gain4/1, "Propeller "/1(rpm)
  "Propeller "/3(eta_p) -> eta_plr/1
  rho/1 -> [rho]
  "Propeller "/1(P_plr (w)) -> Motor/1(P_shaft), Product/1
  rpm_grid/1 -> Motor/6(rpm_grid)
  Gain4/1 -> Product/2  "omega"
  T_y/1 -> Mux2/2
  Mux1/1 -> T_z/1, T_x/1, T_y/1
  T_x/1 -> Mux2/1
  i/1 -> [i]
  T_z/1 -> Mux2/3
  Mux2/1 -> T/1
  [T] -> Mux1/1
  Mux4/1 -> Q/1
  [i] -> Mux3/2
  Q_z/1 -> Mux4/3
  Q_x/1 -> Mux4/1
  Mux3/1 -> Q_z/1, Q_x/1, Q_y/1
  Q_y/1 -> Mux4/2
  [Q] -> Mux3/1
  [i] -> Mux1/2
  Product/1 -> [Q]
  [V] -> Motor/3(V)
  [V] -> "Propeller "/2(V)
  [rho] -> Motor/5(rho)
  [rho] -> "Propeller "/3(rho)
  Constant/1 -> Manual Switch/1
  V/1 -> [V]

== system NumSim_standard_eVTOL/Energy & Power/thrust_3 ==
  note: 将推力、扭矩按电机倾转角转化为向量
  note: 求桨的推力、扭矩、功率、效率
  dt : Inport
  V : Inport  Port=2
  rho : Inport  Port=3
  rpm0 : Inport  Port=4
  rpm_grid : Inport  Port=5
  i : Inport  Port=6
  Constant : Constant  Commented=on  Value=2.5
  Gain4 : Gain  Gain=pi/30
  Manual Switch : ManualSwitch  Commented=on  CurrentSetting=0
  Motor : Subsystem
  Mux1 : Mux  Inputs=2
  Mux2 : Mux  Inputs=3
  Mux3 : Mux  Inputs=2
  Mux4 : Mux  Inputs=3
  Product : Product  Inputs=*/
  "Propeller " : Subsystem
  Q_x : Fcn  Expr=-u[1]*cos(u[2])
  Q_y : Fcn  Expr=0
  Q_z : Fcn  Expr=u[1]*sin(u[2])
  Saturation : Saturate  UpperLimit=inf  LowerLimit=1
  T_x : Fcn  Expr=u[1]*cos(u[2])
  T_y : Fcn  Expr=0
  T_z : Fcn  Expr=-u[1]*sin(u[2])
  eta_plr : Outport  VectorParamsAs1DForOutWhenUnconnected=off
  Q : Outport  Port=2
  T : Outport  Port=3  VectorParamsAs1DForOutWhenUnconnected=off
  rpm : Outport  Port=4  VectorParamsAs1DForOutWhenUnconnected=off
  wires:
  Saturation/1 -> Motor/4(rpm0)
  rpm0/1 -> Saturation/1
  "Propeller "/2(T (N)) -> [T]
  dt/1 -> Motor/2(dt)
  Motor/1(rpm) -> rpm/1, Gain4/1, "Propeller "/1(rpm)
  "Propeller "/3(eta_p) -> eta_plr/1
  rho/1 -> [rho]
  "Propeller "/1(P_plr (w)) -> Motor/1(P_shaft), Product/1
  rpm_grid/1 -> Motor/6(rpm_grid)
  Gain4/1 -> Product/2  "omega"
  T_y/1 -> Mux2/2
  Mux1/1 -> T_z/1, T_x/1, T_y/1
  T_x/1 -> Mux2/1
  i/1 -> [i]
  T_z/1 -> Mux2/3
  Mux2/1 -> T/1
  [T] -> Mux1/1
  Mux4/1 -> Q/1
  [i] -> Mux3/2
  Q_z/1 -> Mux4/3
  Q_x/1 -> Mux4/1
  Mux3/1 -> Q_z/1, Q_x/1, Q_y/1
  Q_y/1 -> Mux4/2
  [Q] -> Mux3/1
  [i] -> Mux1/2
  Product/1 -> [Q]
  [V] -> Motor/3(V)
  [V] -> "Propeller "/2(V)
  [rho] -> Motor/5(rho)
  [rho] -> "Propeller "/3(rho)
  Constant/1 -> Manual Switch/1
  V/1 -> [V]

== system NumSim_standard_eVTOL/Energy & Power/thrust_4 ==
  note: 将推力、扭矩按电机倾转角转化为向量
  note: 求桨的推力、扭矩、功率、效率
  dt : Inport
  V : Inport  Port=2
  rho : Inport  Port=3
  rpm0 : Inport  Port=4
  rpm_grid : Inport  Port=5
  i : Inport  Port=6
  Constant : Constant  Commented=on  Value=2.5
  Gain2 : Gain  Gain=-1
  Gain4 : Gain  Gain=pi/30
  Manual Switch : ManualSwitch  Commented=on  CurrentSetting=0
  Motor : Subsystem
  Mux1 : Mux  Inputs=2
  Mux2 : Mux  Inputs=3
  Mux3 : Mux  Inputs=2
  Mux4 : Mux  Inputs=3
  Product : Product  Inputs=*/
  "Propeller " : Subsystem
  Q_x : Fcn  Expr=-u[1]*cos(u[2])
  Q_y : Fcn  Expr=0
  Q_z : Fcn  Expr=u[1]*sin(u[2])
  Saturation : Saturate  UpperLimit=inf  LowerLimit=1
  T_x : Fcn  Expr=u[1]*cos(u[2])
  T_y : Fcn  Expr=0
  T_z : Fcn  Expr=-u[1]*sin(u[2])
  eta_plr : Outport  VectorParamsAs1DForOutWhenUnconnected=off
  Q : Outport  Port=2
  T : Outport  Port=3  VectorParamsAs1DForOutWhenUnconnected=off
  rpm : Outport  Port=4  VectorParamsAs1DForOutWhenUnconnected=off
  wires:
  Saturation/1 -> Motor/4(rpm0)
  rpm0/1 -> Saturation/1
  "Propeller "/2(T (N)) -> [T]
  dt/1 -> Motor/2(dt)
  Motor/1(rpm) -> rpm/1, Gain4/1, "Propeller "/1(rpm)
  "Propeller "/3(eta_p) -> eta_plr/1
  rho/1 -> [rho]
  "Propeller "/1(P_plr (w)) -> Motor/1(P_shaft), Product/1
  rpm_grid/1 -> Motor/6(rpm_grid)
  Gain4/1 -> Product/2  "omega"
  T_y/1 -> Mux2/2
  Mux1/1 -> T_z/1, T_x/1, T_y/1
  T_x/1 -> Mux2/1
  i/1 -> [i]
  T_z/1 -> Mux2/3
  Mux2/1 -> T/1
  [T] -> Mux1/1
  Mux4/1 -> Q/1
  [i] -> Mux3/2
  Q_z/1 -> Mux4/3
  Q_x/1 -> Mux4/1
  Mux3/1 -> Q_z/1, Q_x/1, Q_y/1
  Q_y/1 -> Mux4/2
  [Q] -> Mux3/1
  [i] -> Mux1/2
  Product/1 -> Gain2/1
  [V] -> Motor/3(V)
  [V] -> "Propeller "/2(V)
  [rho] -> Motor/5(rho)
  [rho] -> "Propeller "/3(rho)
  Gain2/1 -> [Q]
  Constant/1 -> Manual Switch/1
  V/1 -> [V]

== system NumSim_standard_eVTOL/Energy & Power/thrust_5 ==
  note: 将推力、扭矩按电机倾转角转化为向量
  note: 求桨的推力、扭矩、功率、效率
  dt : Inport
  V : Inport  Port=2
  rho : Inport  Port=3
  rpm0 : Inport  Port=4
  rpm_grid : Inport  Port=5
  i : Inport  Port=6
  Constant : Constant  Commented=on  Value=2.5
  Gain2 : Gain  Gain=-1
  Gain4 : Gain  Gain=pi/30
  Manual Switch : ManualSwitch  Commented=on  CurrentSetting=0
  Motor : Subsystem
  Mux1 : Mux  Inputs=2
  Mux2 : Mux  Inputs=3
  Mux3 : Mux  Inputs=2
  Mux4 : Mux  Inputs=3
  Product : Product  Inputs=*/
  "Propeller " : Subsystem
  Q_x : Fcn  Expr=-u[1]*cos(u[2])
  Q_y : Fcn  Expr=0
  Q_z : Fcn  Expr=u[1]*sin(u[2])
  Saturation : Saturate  UpperLimit=inf  LowerLimit=1
  T_x : Fcn  Expr=u[1]*cos(u[2])
  T_y : Fcn  Expr=0
  T_z : Fcn  Expr=-u[1]*sin(u[2])
  eta_plr : Outport  VectorParamsAs1DForOutWhenUnconnected=off
  Q : Outport  Port=2
  T : Outport  Port=3  VectorParamsAs1DForOutWhenUnconnected=off
  rpm : Outport  Port=4  VectorParamsAs1DForOutWhenUnconnected=off
  wires:
  Saturation/1 -> Motor/4(rpm0)
  rpm0/1 -> Saturation/1
  "Propeller "/2(T (N)) -> [T]
  dt/1 -> Motor/2(dt)
  Motor/1(rpm) -> rpm/1, Gain4/1, "Propeller "/1(rpm)
  "Propeller "/3(eta_p) -> eta_plr/1
  rho/1 -> [rho]
  "Propeller "/1(P_plr (w)) -> Motor/1(P_shaft), Product/1
  rpm_grid/1 -> Motor/6(rpm_grid)
  Gain4/1 -> Product/2  "omega"
  T_y/1 -> Mux2/2
  Mux1/1 -> T_z/1, T_x/1, T_y/1
  T_x/1 -> Mux2/1
  i/1 -> [i]
  T_z/1 -> Mux2/3
  Mux2/1 -> T/1
  [T] -> Mux1/1
  Mux4/1 -> Q/1
  [i] -> Mux3/2
  Q_z/1 -> Mux4/3
  Q_x/1 -> Mux4/1
  Mux3/1 -> Q_z/1, Q_x/1, Q_y/1
  Q_y/1 -> Mux4/2
  [Q] -> Mux3/1
  [i] -> Mux1/2
  Product/1 -> Gain2/1
  [V] -> Motor/3(V)
  [V] -> "Propeller "/2(V)
  [rho] -> Motor/5(rho)
  [rho] -> "Propeller "/3(rho)
  Gain2/1 -> [Q]
  Constant/1 -> Manual Switch/1
  V/1 -> [V]

== system NumSim_standard_eVTOL/Energy & Power/thrust_6 ==
  note: 将推力、扭矩按电机倾转角转化为向量
  note: 求桨的推力、扭矩、功率、效率
  dt : Inport
  V : Inport  Port=2
  rho : Inport  Port=3
  rpm0 : Inport  Port=4
  rpm_grid : Inport  Port=5
  i : Inport  Port=6
  Constant : Constant  Commented=on  Value=2.5
  Gain4 : Gain  Gain=pi/30
  Manual Switch : ManualSwitch  Commented=on  CurrentSetting=0
  Motor : Subsystem
  Mux1 : Mux  Inputs=2
  Mux2 : Mux  Inputs=3
  Mux3 : Mux  Inputs=2
  Mux4 : Mux  Inputs=3
  Product : Product  Inputs=*/
  "Propeller " : Subsystem
  Q_x : Fcn  Expr=-u[1]*cos(u[2])
  Q_y : Fcn  Expr=0
  Q_z : Fcn  Expr=u[1]*sin(u[2])
  Saturation : Saturate  UpperLimit=inf  LowerLimit=1
  T_x : Fcn  Expr=u[1]*cos(u[2])
  T_y : Fcn  Expr=0
  T_z : Fcn  Expr=-u[1]*sin(u[2])
  eta_plr : Outport  VectorParamsAs1DForOutWhenUnconnected=off
  Q : Outport  Port=2
  T : Outport  Port=3  VectorParamsAs1DForOutWhenUnconnected=off
  rpm : Outport  Port=4  VectorParamsAs1DForOutWhenUnconnected=off
  wires:
  Saturation/1 -> Motor/4(rpm0)
  rpm0/1 -> Saturation/1
  "Propeller "/2(T (N)) -> [T]
  dt/1 -> Motor/2(dt)
  Motor/1(rpm) -> rpm/1, Gain4/1, "Propeller "/1(rpm)
  "Propeller "/3(eta_p) -> eta_plr/1
  rho/1 -> [rho]
  "Propeller "/1(P_plr (w)) -> Motor/1(P_shaft), Product/1
  rpm_grid/1 -> Motor/6(rpm_grid)
  Gain4/1 -> Product/2  "omega"
  T_y/1 -> Mux2/2
  Mux1/1 -> T_z/1, T_x/1, T_y/1
  T_x/1 -> Mux2/1
  i/1 -> [i]
  T_z/1 -> Mux2/3
  Mux2/1 -> T/1
  [T] -> Mux1/1
  Mux4/1 -> Q/1
  [i] -> Mux3/2
  Q_z/1 -> Mux4/3
  Q_x/1 -> Mux4/1
  Mux3/1 -> Q_z/1, Q_x/1, Q_y/1
  Q_y/1 -> Mux4/2
  [Q] -> Mux3/1
  [i] -> Mux1/2
  [V] -> Motor/3(V)
  [V] -> "Propeller "/2(V)
  [rho] -> Motor/5(rho)
  [rho] -> "Propeller "/3(rho)
  Product/1 -> [Q]
  Constant/1 -> Manual Switch/1
  V/1 -> [V]

== system NumSim_standard_eVTOL/Environment/Terrain ==
  Xe : Inport
  Terminator : Terminator
  hground_value : Constant  OutDataTypeStr=single
  hground : Outport  VectorParamsAs1DForOutWhenUnconnected=off
  wires:
  Xe/1 -> Terminator/1
  hground_value/1 -> hground/1  "hground"

== system NumSim_standard_eVTOL/Environment/Wind Models ==
  Xe_x : Inport
  Ve : Inport  Port=2
  Altitude : Inport  Port=3
  DCM : Inport  Port=4
  Constant1 : Constant  Value=[0,0,0]
  Constant2 : Constant  Value=[0,0,0]
  Dot Product1 : DotProduct  OutDataTypeStr=Inherit: Inherit via internal rule
  Dot Product2 : DotProduct  OutDataTypeStr=Inherit: Inherit via internal rule
  Dryden Wind Turbulence Model (Continuous (+q -r)) : Subsystem  AncestorBlock=|  mask(Wind Turbulence Model){units=Metric (MKS), spec=MIL-F-8785C, model=Continuous Dryden (+q -r), W20=8, Wdeg=0, TurbProb=10^-4, L_high=533.4, Wingspan=7, ts=0.01, Seed=[23341 23342 23343 23344], T_on=on}
      | CustomLib_2019b/Dryden Wind Turbulence Model 
      | (Continuous (+q -r))
      mask prompts: units "aeroblks:aeroblkwind:blockWindTurbulenceModelParamUnits"; spec "aeroblks:aeroblkwind:blockWindTurbulenceModelParamSpecification"; model "aeroblks:aeroblkwind:blockWindTurbulenceModelParamModeltype"; W20 "Wind speed at 6 m defines the low-altitude intensity (m/s):"; Wdeg "Wind direction at 6 m (degrees clockwise from north):"; TurbProb "aeroblks:aeroblkwind:blockWindTurbulenceModelParamProbabilityofexceedanceofhighaltitudeintensity"; L_high "Scale length at medium/high altitudes (m):"; Wingspan "Wingspan (m):"; ts "Band limited noise sample time (sec):"; Seed "aeroblks:aeroblkwind:blockWindTurbulenceModelParamNoiseseedsugvgwgpg"; T_on "aeroblks:aeroblkwind:blockWindTurbulenceModelParamTurbulenceon"
      mask help: aeroblks:aeroblkwind:blockWindTurbulenceModelDesc
      mask init:
      | index = strfind(model,' ');
      | disp1 = model(1:index(1)-1);
      | disp2 = model(index(1)+1:index(end-1)-1);
      | disp3 = model(index(end-1)+1:end);
      | 
      | h_vec = [.5 1.75 3.75 7.5 15 25 35 45 55 65 75 80]*1000;% feet
      | sigma_vec(1,:) = [3.2 2.2 1.5 zeros(1,9)]; % ft/sec
      | sigma_vec(2,:) = [4.2 3.6 3.3 1.6 zeros(1,8)];
      | sigma_vec(3,:) = [6.6 6.9 7.4 6.7 4.6 2.7 0.4 zeros(1,5)];
      | sigma_vec(4,:) = [8.6 9.6 10.6 10.1 8.0 6.6 5.0 4.2 2.7 zeros(1,3)];
      | sigma_vec(5,:) = [11.8 13.0 16.0 15.1 11.6 9.7 8.1 8.2 7.9 4.9 3.2 2.1];
      | sigma_vec(6,:) = [15.6 17.6 23.0 23.6 22.1 20.0 16.0 15.1 12.1 7.9 6.2 5.1];
      | sigma_vec(7,:) = [18.7 21.5 28.4 30.2 30.7 31.0 25.2 23.1 17.5 10.7 8.4 7.2];
      | max_height_low = 1000;
      | if strcmp(spec,'MIL-F-8785C')
      |     min_height_high = 2000;
      | else
      | 	min_height_high = 1750;
      | end
      | [ports] = aeroicon('aeroblkwindturb2','icon');
      | 
      | dt=ts;
      settings: LibrarySourceBlock=|
      | CustomLib_2019b/Dryden Wind Turbulence Model
      | (Continuous (+q -r))
      mask Help: eval('asbhelp(''Dryden Wind Turbulence Model (Continuous)'')');
      mask TypeOptions units: aeroblks:aeroblkwind:blockWindTurbulenceModelParamComboMetricMKS | aeroblks:aeroblkwind:blockWindTurbulenceModelParamComboEnglishVelocityinfts | aeroblks:aeroblkwind:blockWindTurbulenceModelParamComboEnglishVelocityinkts
      mask TypeOptions spec: aeroblks:aeroblkwind:blockWindTurbulenceModelParamComboMILF8785C | aeroblks:aeroblkwind:blockWindTurbulenceModelParamComboMILHDBK1797 | aeroblks:aeroblkwind:blockWindTurbulenceModelParamComboMILHDBK1797B
      mask TypeOptions model: aeroblks:aeroblkwind:blockWindTurbulenceModelParamComboContinuousVonKarmanqr1 | aeroblks:aeroblkwind:blockWindTurbulenceModelParamComboContinuousVonKarmanqr2 | aeroblks:aeroblkwind:blockWindTurbulenceModelParamComboContinuousVonKarmanqr3 | aeroblks:aeroblkwind:blockWindTurbulenceModelParamComboContinuousDrydenqr1 | aeroblks:aeroblkwind:blockWindTurbulenceModelParamComboContinuousDrydenqr2 | aeroblks:aeroblkwind:blockWindTurbulenceModelParamComboContinuousDrydenqr3 | aeroblks:aeroblkwind:blockWindTurbulenceModelParamComboDiscreteDrydenqr1 | aeroblks:aeroblkwind:blockWindTurbulenceModelParamComboDiscreteDrydenqr2 | aeroblks:aeroblkwind:blockWindTurbulenceModelParamComboDiscreteDrydenqr3
      mask Callback model: aeroicon('aeroblkwindturb2');
      mask TypeOptions TurbProb: aeroblks:aeroblkwind:blockWindTurbulenceModelParamCombo2x101 | aeroblks:aeroblkwind:blockWindTurbulenceModelParamCombo101 | aeroblks:aeroblkwind:blockWindTurbulenceModelParamCombo102Light | aeroblks:aeroblkwind:blockWindTurbulenceModelParamCombo103Moderate | aeroblks:aeroblkwind:blockWindTurbulenceModelParamCombo104 | aeroblks:aeroblkwind:blockWindTurbulenceModelParamCombo105Severe | aeroblks:aeroblkwind:blockWindTurbulenceModelParamCombo106
      mask DialogControl units Prompt: Units:
      mask DialogControl spec Prompt: Specification:
      mask DialogControl model Prompt: Model type:
      mask DialogControl TurbProb Prompt: Probability of exceedance of high-altitude intensity:
      mask DialogControl Seed Prompt: Noise seeds [ug vg wg pg]:
      mask DialogControl T_on Prompt: Turbulence on
      mask Display:
      | port_label(ports(1).type,ports(1).port,ports(1).txt,'texmode','on');
      | port_label(ports(2).type,ports(2).port,ports(2).txt,'texmode','on');
      | port_label(ports(3).type,ports(3).port,ports(3).txt,'texmode','on');
      | port_label(ports(4).type,ports(4).port,ports(4).txt,'texmode','on');
      | port_label(ports(5).type,ports(5).port,ports(5).txt,'texmode','on');
  Gain4 : Gain  Gain=[1,1,1]
  Manual Switch1 : ManualSwitch  CurrentSetting=0
  Manual Switch2 : ManualSwitch  CurrentSetting=0
  Sqrt : Sqrt
  vt1 : Math  Operator=sqrt  SignedPower=on
  wind scp2 : Scope
  wind_mag scp : Scope
  windangular scp : Scope
  windspeed scp : Scope
  ug,vg,wg1 : Outport  VectorParamsAs1DForOutWhenUnconnected=off
  pg,qg,rg1 : Outport  Port=2  VectorParamsAs1DForOutWhenUnconnected=off
  wires:
  Manual Switch2/1 -> ug,vg,wg1/1  "WindVelocity"
  Dryden Wind Turbulence Model (Continuous (+q -r))/1(ug,vg,wg) -> Gain4/1, windspeed scp/1, Dot Product2/2, Dot Product2/1  "Vw"
  Dryden Wind Turbulence Model (Continuous (+q -r))/2(pg,qg,rg) -> Manual Switch1/1, windangular scp/1  "WindAngularRates"
  Constant1/1 -> Manual Switch1/2
  Altitude/1 -> [Altitude]
  vt1/1 -> [Airspeed]  "Airspeed"
  Constant2/1 -> Manual Switch2/2
  [Airspeed] -> Dryden Wind Turbulence Model (Continuous (+q -r))/2(Airspeed)  "Airspeed"
  DCM/1 -> [DCM]
  Ve/1 -> Dot Product1/2, Dot Product1/1
  Manual Switch1/1 -> pg,qg,rg1/1  "WindAngularRates"
  Gain4/1 -> Manual Switch2/1  "WindVelocity"
  [Altitude] -> Dryden Wind Turbulence Model (Continuous (+q -r))/1(Altitude)
  Dot Product2/1 -> Sqrt/1
  [DCM] -> Dryden Wind Turbulence Model (Continuous (+q -r))/3(DCM)
  Dot Product1/1 -> vt1/1
  Sqrt/1 -> wind_mag scp/1  "wind_mag"
  Xe_x/1 -> [x]
  [x] -> wind scp2/1
